simulink model "ME322_Exercise_3_Prelab_Simulink"  (R2024b)
settings: Solver=VariableStepAuto  StartTime=0.0  StopTime=10.0  RelTol=1e-3
undefined symbols (not defined in the file): b, k, m
settings Model: Creator=Caide  LastModifiedBy=Caide

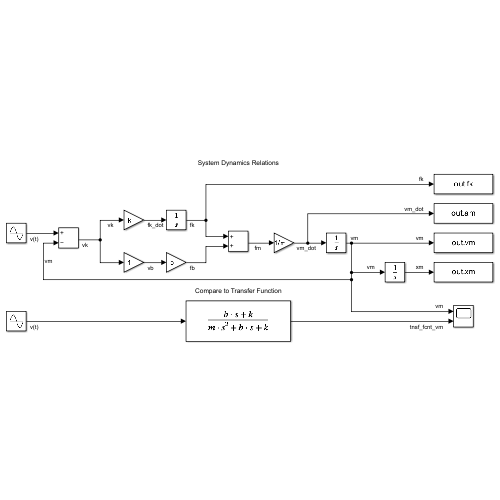
[thumbnail: Simulink's stored preview of the top-level diagram]
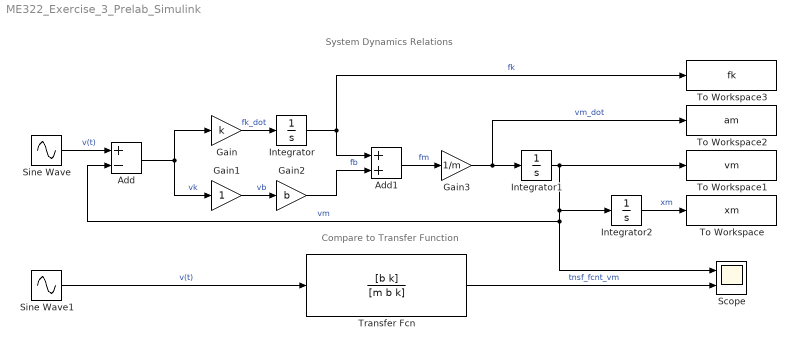
== system ME322_Exercise_3_Prelab_Simulink ==
  note: Compare to Transfer Function
  note: System Dynamics Relations
  Add : Sum  Inputs=+-
  Add1 : Sum
  Gain : Gain  Gain=k
  Gain1 : Gain
  Gain2 : Gain  Gain=b
  Gain3 : Gain  Gain=1/m
  Integrator : Integrator
  Integrator1 : Integrator
  Integrator2 : Integrator
  Scope : Scope  NumInputPorts=2
  Sine Wave : Sin  Amplitude=5  SampleTime=0
  Sine Wave1 : Sin  Amplitude=5  SampleTime=0
  To Workspace : ToWorkspace  VariableName=xm  SampleTime=-1
  To Workspace1 : ToWorkspace  VariableName=vm  SampleTime=-1
  To Workspace2 : ToWorkspace  VariableName=am  SampleTime=-1
  To Workspace3 : ToWorkspace  VariableName=fk  SampleTime=-1
  Transfer Fcn : TransferFcn  Numerator=[b k]  Denominator=[m b k]
  wires:
  Sine Wave/1 -> Add/1  "v(t)"
  Add/1 -> Gain/1, Gain1/1  "vk"
  Gain2/1 -> Add1/2  "fb"
  Gain3/1 -> Integrator1/1, To Workspace2/1  "vm_dot"
  Gain/1 -> Integrator/1  "fk_dot"
  Integrator/1 -> To Workspace3/1, Add1/1  "fk"
  Add1/1 -> Gain3/1  "fm"
  Gain1/1 -> Gain2/1  "vb"
  Integrator2/1 -> To Workspace/1  "xm"
  Integrator1/1 -> To Workspace1/1, Integrator2/1, Scope/1, Add/2  "vm"
  Sine Wave1/1 -> Transfer Fcn/1  "v(t)"
  Transfer Fcn/1 -> Scope/2  "tnsf_fcnt_vm"
